simulink model "abs_EV"  (R2023a)
settings: Solver=ode45  StartTime=0  StopTime=15  FixedStep=0.002  RelTol=1e-3  AbsTol=1e-6
libraries: cstblocks x2, simulink x2, Solver_SF x1
settings Model: ExtModeTrigMode=oneshot  VariantFading=off  Creator=ywata  LastModifiedBy=USER
settings SolverCC: AutoScaleAbsTol=off  AlgebraicLoopSolver=TrustRegion
settings DataIOCC: SaveFormat=Array  SignalLoggingSaveFormat=ModelDataLogs  ReturnWorkspaceOutputs=off  SignalLoggingName=sigsOut
settings OptimizationCC: BlockReduction=off  BooleanDataType=off  ExpressionDepthLimit=2147483647  LifeSpan=inf
settings DebuggingCC: SaveWithParameterizedLinksMsg=none  UnderspecifiedInitializationDetection=Classic  MergeDetectMultiDrivingBlocksExec=none  SignalResolutionControl=TryResolveAllWithWarning  MultiTaskDSMMsg=warning  MultiTaskCondExecSysMsg=none  FcnCallInpInsideContextMsg=warning  UnconnectedInputMsg=warning  UnconnectedOutputMsg=warning  UnconnectedLineMsg=warning  StateNameClashWarn=warning  SFUnexpectedBacktrackingDiag=warning  SFNoUnconditionalDefaultTransitionDiag=warning  SFExecutionAtInitializationDiag=none  ArithmeticOperatorsInVariantConditions=warning
settings HardwareCC: ProdBitPerPointer=32  ProdBitPerSizeT=32  ProdBitPerPtrDiffT=32  ProdLargestAtomicFloat=None  ProdIntDivRoundTo=Undefined  ProdEndianess=Unspecified  ProdWordSize=32  ProdHWDeviceType=32-bit Generic  TargetUnknown=on
settings ModelReferenceCC: PropagateSignalLabelsOutOfModel=off
settings SFSimCC: SimUseLocalCustomCode=off  CustomCodeUndefinedFunction=UseInterfaceOnly
settings RTWCC: TemplateMakefile=grt_vc.tmf  RTWUseLocalCustomCode=off
settings CodeAppCC: StateflowObjectComments=on
settings GRTTargetCC: TargetFcnLib=ansi_tfl_tmw.mat  TargetLangStandard=C89/C90 (ANSI)  CombineOutputUpdateFcns=off  GRTInterface=on
settings ConfigComp: CovMetricSettings=dw  CovSaveCumulativeToWorkspaceVar=on  CovSaveSingleToWorkspaceVar=on  CovExternalEMLEnable=off

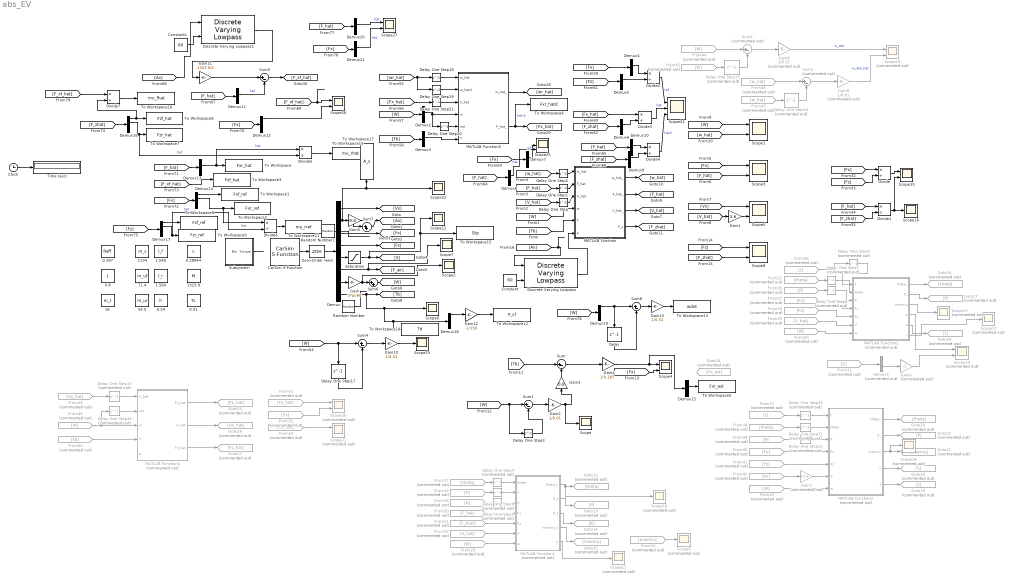
== system abs_EV ==
  0.01 : DataStoreMemory  DataStoreName=Ts  WriteAfterWriteMsg=warning  InitialValue=0.01  ShowAdditionalParam=off  OutDataTypeStr=double
  0.287 : DataStoreMemory  DataStoreName=Reff  WriteAfterWriteMsg=warning  InitialValue=0.287  ShowAdditionalParam=off  OutDataTypeStr=double
  0.28944 : DataStoreMemory  DataStoreName=c  WriteAfterWriteMsg=warning  InitialValue=0.29844  ShowAdditionalParam=off  OutDataTypeStr=double
  0.54 : DataStoreMemory  DataStoreName=h  WriteAfterWriteMsg=warning  InitialValue=0.54  ShowAdditionalParam=off  OutDataTypeStr=double
  0.8 : DataStoreMemory  DataStoreName=J  WriteAfterWriteMsg=warning  InitialValue=0.8  ShowAdditionalParam=off  OutDataTypeStr=double
  1.040 : DataStoreMemory  DataStoreName=l_f  WriteAfterWriteMsg=warning  InitialValue=1.040  ShowAdditionalParam=off  OutDataTypeStr=double
  1.560 : DataStoreMemory  DataStoreName=l_r  WriteAfterWriteMsg=warning  InitialValue=1.560  ShowAdditionalParam=off  OutDataTypeStr=double
  1134 : DataStoreMemory  DataStoreName=m_s  WriteAfterWriteMsg=warning  InitialValue=1134  ShowAdditionalParam=off  OutDataTypeStr=double
  1323.9 : DataStoreMemory  DataStoreName=M  WriteAfterWriteMsg=warning  InitialValue=1323.9  ShowAdditionalParam=off  OutDataTypeStr=double
  16 : DataStoreMemory  DataStoreName=m_t  WriteAfterWriteMsg=warning  InitialValue=16  ShowAdditionalParam=off  OutDataTypeStr=double
  54.5 : DataStoreMemory  DataStoreName=m_ur  WriteAfterWriteMsg=warning  InitialValue=54.5  ShowAdditionalParam=off  OutDataTypeStr=double
  71.4 : DataStoreMemory  DataStoreName=m_uf  WriteAfterWriteMsg=warning  InitialValue=71.4  ShowAdditionalParam=off  OutDataTypeStr=double
  CarSim S-Function : Solver_SF/CarSim S-Function  Priority=1  SIMFILE=simfile.sim  Run_RTs=off  vs_state_ind=Run  StopMode_ind=Vehicle Model
  Clock : Clock
  Constant : Constant  Value=60
  Constant1 : Constant  Value=60
  Delay : Delay  DelayLength=1  InitialCondition=67.655
  Delay One Step : Delay  DelayLength=1  InitialCondition=19.444
  Delay One Step1 : Delay  DelayLength=1  InitialCondition=[0 0 0 0]'
  Delay One Step10 : Delay  Commented=on  DelayLength=1
  Delay One Step11 : Delay  Commented=on  DelayLength=1  InitialCondition=[0 0]'
  Delay One Step12 : Delay  Commented=on  DelayLength=1  InitialCondition=[0 0;0 0]
  Delay One Step13 : Delay  Commented=on  DelayLength=1
  Delay One Step14 : Delay  Commented=on  DelayLength=1
  Delay One Step15 : Delay  Commented=on  DelayLength=1  InitialCondition=70/3.6
  Delay One Step16 : Delay  Commented=on  DelayLength=1  InitialCondition=67.75*ones(4,1)
  Delay One Step17 : Delay  DelayLength=1  InitialCondition=70/3.6/0.287
  Delay One Step18 : Delay  DelayLength=1  InitialCondition=67.655
  Delay One Step19 : Delay  InitialCondition=67.655
  Delay One Step2 : Delay  DelayLength=1  InitialCondition=[67.655 67.655 67.655 67.655]'
  Delay One Step20 : Delay  DelayLength=1  InitialCondition=67.655
  Delay One Step21 : Delay  DelayLength=1  InitialCondition=0
  Delay One Step3 : Delay  DelayLength=1  InitialCondition=[67.655 67.655 67.655 67.655]'
  Delay One Step4 : Delay  Commented=on  DelayLength=1  InitialCondition=ones(2,4)
  Delay One Step5 : Delay  Commented=on  DelayLength=1  InitialCondition=0.1*ones(2,4)
  Delay One Step6 : Delay  Commented=on  DelayLength=1  InitialCondition=0.1*ones(2,8)
  Delay One Step7 : Delay  Commented=on  DelayLength=1  InitialCondition=[300;0.1]
  Delay One Step8 : Delay  Commented=on  DelayLength=1  InitialCondition=[3 0;0 0.001]
  Delay One Step9 : Delay  Commented=on  DelayLength=1  InitialCondition=0
  Demux : Demux  Outputs=[1 1 4 4 4 1 4 4]
  Demux1 : Demux  Commented=on
  Demux{2..21} (20 alike) : Demux
  Discrete Varying Lowpass : cstblocks/Linear Parameter Varying/Discrete Varying Lowpass  N=1  w0=0  Ts=0.01
  Discrete Varying Lowpass1 : cstblocks/Linear Parameter Varying/Discrete Varying Lowpass  N=1  w0=0  Ts=0.01
  Divide{,1..7} (8 alike) : Product  Inputs=*/
  From17 : From  Commented=on  GotoTag=theta
  From18 : From  Commented=on  GotoTag=K
  From19 : From  Commented=on  GotoTag=P
  From20 : From  Commented=on  GotoTag=F_hat
  From21 : From  Commented=on  GotoTag=F_zhat
  From22 : From  Commented=on  GotoTag=V_hat
  From{23,30,43..45,49} (6 alike) : From  Commented=on  GotoTag=W
  From24 : From  Commented=on  GotoTag=maxmu
  From25 : From  Commented=on  GotoTag=theta
  From26 : From  Commented=on  GotoTag=P
  From27 : From  Commented=on  GotoTag=Fx
  From28 : From  Commented=on  GotoTag=Fz
  From29 : From  Commented=on  GotoTag=V_hat
  From31 : From  Commented=on  GotoTag=S
  From36 : From  Commented=on  GotoTag=t
  From37 : From  Commented=on  GotoTag=t
  From38 : From  Commented=on  GotoTag=theta
  From39 : From  Commented=on  GotoTag=P
  From40 : From  Commented=on  GotoTag=Fx
  From41 : From  Commented=on  GotoTag=Fz
  From42 : From  Commented=on  GotoTag=Vx
  From46 : From  Commented=on  GotoTag=w_hat
  From47 : From  Commented=on  GotoTag=w_hat
  From48 : From  Commented=on  GotoTag=Vx_hat
  From50 : From  Commented=on  GotoTag=Tb
  From51 : From  Commented=on  GotoTag=Fx_hat
  From52 : From  Commented=on  GotoTag=Fx
  From53 : From  Commented=on  GotoTag=Vx_hat
  Gain : Gain  Gain=2*pi/60
  Gain1 : Gain  Gain=3.6
  Gain10 : Gain  Gain=1/0.01
  Gain11 : Gain  Gain=1323.9/2
  Gain12 : Gain  Gain=-1/150
  Gain13 : Gain  Gain=1/0.01
  Gain2 : Gain  Gain=1/0.01
  Gain3 : Gain  Gain=0.8
  Gain4 : Gain  Gain=1/0.287
  Gain5 : Gain  Gain=9.8
  Gain6 : Gain  Commented=on  Gain=-1
  Gain7 : Gain  Commented=on  Gain=1/3.6
  Gain8 : Gain  Commented=on  Gain=1/0.01
  Gain9 : Gain  Commented=on  Gain=1/0.01
  Goto12 : Goto  Commented=on  GotoTag=theta
  Goto13 : Goto  Commented=on  GotoTag=P
  Goto14 : Goto  Commented=on  GotoTag=K
  Goto15 : Goto  Commented=on  GotoTag=maxmu
  Goto16 : Goto  Commented=on  GotoTag=theta
  Goto17 : Goto  Commented=on  GotoTag=P
  Goto18 : Goto  Commented=on  GotoTag=t
  Goto19 : Goto  Commented=on  GotoTag=t
  Goto20 : Goto  Commented=on  GotoTag=s
  Goto21 : Goto  Commented=on  GotoTag=maxmu
  Goto22 : Goto  Commented=on  GotoTag=P
  Goto23 : Goto  Commented=on  GotoTag=theta
  Goto24 : Goto  Commented=on  GotoTag=Fx_est
  Goto25 : Goto  Commented=on  GotoTag=Fx_hat
  Goto26 : Goto  Commented=on  GotoTag=Vx_hat
  Goto27 : Goto  Commented=on  GotoTag=Fz_hat
  MATLAB Function : MATLAB Function  TreatAsAtomicUnit=on
  MATLAB Function1 : MATLAB Function  Commented=on  TreatAsAtomicUnit=on
  MATLAB Function2 : MATLAB Function  Commented=on  TreatAsAtomicUnit=on
  MATLAB Function3 : MATLAB Function  Commented=on  TreatAsAtomicUnit=on
  MATLAB Function4 : MATLAB Function  Commented=on  TreatAsAtomicUnit=on
  MATLAB Function5 : MATLAB Function  TreatAsAtomicUnit=on
  Random Number : RandomNumber  Variance=0.01^2  SampleTime=0.01
  Random Number1 : RandomNumber  Variance=0.01  SampleTime=0.01
  Saturation : Saturate  UpperLimit=1  LowerLimit=-1
  Scope{,2,6..7,12,16,22..23} (8 alike) : Scope
  Scope{1,3..5,8,15,26..27} (8 alike) : Scope  NumInputPorts=2
  Scope{9..11,13,17..18} (6 alike) : Scope  Commented=on
  Scope{14,19..21} (4 alike) : Scope  Commented=on  NumInputPorts=2
  Scope24 : Scope  NumInputPorts=3
  Scope25 : Scope  NumInputPorts=3
  Subsystem : Subsystem
  Sum{,1,4..5,8} (5 alike) : Sum  Inputs=|+-
  Sum2 : Sum  Commented=on  Inputs=|+-
  Sum3 : Sum  Commented=on  Inputs=|+-
  Sum6 : Sum  Inputs=|++
  Sum7 : Sum  Inputs=|++
  Time (sec) : Display
      settings: Format=bank  Decimation=100
  To Workspace : ToWorkspace  VariableName=Fxr_hat  SaveFormat=Timeseries  SampleTime=-1
  To Workspace1 : ToWorkspace  VariableName=Fxf_ref  SaveFormat=Timeseries  SampleTime=-1
  To Workspace10 : ToWorkspace  VariableName=mu_rhat  SaveFormat=Timeseries  SampleTime=-1
  To Workspace11 : ToWorkspace  VariableName=mu_rref  SaveFormat=Timeseries  SampleTime=-1
  To Workspace12 : ToWorkspace  VariableName=P_cf  SaveFormat=Timeseries  SampleTime=-1
  To Workspace13 : ToWorkspace  VariableName=wdot  SaveFormat=Timeseries  SampleTime=-1
  To Workspace14 : ToWorkspace  VariableName=Td  SaveFormat=Timeseries  SampleTime=-1
  To Workspace15 : ToWorkspace  VariableName=Slip  SaveFormat=Timeseries  SampleTime=-1
  To Workspace16 : ToWorkspace  VariableName=mu_fhat  SaveFormat=Timeseries  SampleTime=-1
  To Workspace17 : ToWorkspace  VariableName=A_x  SaveFormat=Timeseries  SampleTime=-1
  To Workspace2 : ToWorkspace  VariableName=Fxr_ref  SaveFormat=Timeseries  SampleTime=-1
  To Workspace3 : ToWorkspace  VariableName=Fxf_hat  SaveFormat=Timeseries  SampleTime=-1
  To Workspace4 : ToWorkspace  VariableName=Fxr_hatd  SaveFormat=Timeseries  SampleTime=-1
  To Workspace5 : ToWorkspace  VariableName=Fxr_est  SaveFormat=Timeseries  SampleTime=-1
  To Workspace6 : ToWorkspace  VariableName=Fzf_hat  SaveFormat=Timeseries  SampleTime=-1
  To Workspace7 : ToWorkspace  VariableName=Fzr_hat  SaveFormat=Timeseries  SampleTime=-1
  To Workspace8 : ToWorkspace  VariableName=Fzf_ref  SaveFormat=Timeseries  SampleTime=-1
  To Workspace9 : ToWorkspace  VariableName=Fzr_ref  SaveFormat=Timeseries  SampleTime=-1
  Zero-Order Hold : ZeroOrderHold  SampleTime=0.01
  wires:
  CarSim S-Function/1 -> Zero-Order Hold/1
  Clock/1 -> Time (sec)/1
  Demux/1 -> [Vx]
  Demux/3 -> [Fx]
  Demux/4 -> [Fz]
  Demux/7 -> Gain/1
  Gain/1 -> Scope2/1, Sum6/1
  Demux/8 -> To Workspace14/1, Demux18/1, Scope6/1, [Tb]
  Zero-Order Hold/1 -> Demux/1
  [Tb] -> MATLAB Function/5(T)
  [W] -> MATLAB Function/4(w)
  MATLAB Function/3(V_hat_) -> [V_hat]
  MATLAB Function/2(F_hat_) -> [F_hat]
  MATLAB Function/1(w_hat_) -> [w_hat]
  [V_hat] -> Delay One Step/1
  Delay One Step/1 -> MATLAB Function/3(V_hat)
  [F_hat] -> Delay One Step1/1
  Delay One Step1/1 -> MATLAB Function/2(F_hat)
  [w_hat] -> Delay One Step2/1
  Delay One Step2/1 -> MATLAB Function/1(w_hat)
  [Fx] -> Scope3/1
  [F_hat] -> Scope3/2
  [V_hat] -> Gain1/1
  [Vx] -> Scope5/1
  Gain1/1 -> Scope5/2
  [W] -> Scope1/1
  [w_hat] -> Scope1/2
  [Tb] -> Sum/1
  [W] -> Delay One Step3/1, Sum1/1
  Delay One Step3/1 -> Sum1/2
  Gain2/1 -> Scope/1, Gain3/1
  Gain3/1 -> Sum/2
  Sum/1 -> Gain4/1
  Gain4/1 -> Demux15/1, Scope4/1
  [Fx] -> Scope4/2
  Sum1/1 -> Gain2/1
  Demux/6 -> Scope7/1, [F_air]
  MATLAB Function/4(F_z) -> [F_zhat]
  [F_zhat] -> Scope8/2
  [Fz] -> Scope8/1
  [Ax] -> Discrete Varying Lowpass/1
  Gain5/1 -> Sum7/1
  MATLAB Function1/1(theta_t) -> Scope10/1, Goto12/1
  MATLAB Function1/2(P_t) -> Goto13/1
  MATLAB Function1/3(K_t) -> Goto14/1
  MATLAB Function1/4(maxmu_t) -> Goto15/1
  From17/1 -> Delay One Step4/1
  Delay One Step4/1 -> MATLAB Function1/1(theta)
  From18/1 -> Delay One Step5/1
  Delay One Step5/1 -> MATLAB Function1/3(K)
  From19/1 -> Delay One Step6/1
  Delay One Step6/1 -> MATLAB Function1/2(P)
  From20/1 -> MATLAB Function1/4(Fx)
  From21/1 -> MATLAB Function1/5(Fz)
  From22/1 -> MATLAB Function1/6(V)
  From23/1 -> MATLAB Function1/7(w)
  From24/1 -> Scope9/1
  MATLAB Function1/5(s) -> Scope11/1
  From25/1 -> Delay One Step7/1
  Delay One Step7/1 -> MATLAB Function2/2(theta)
  Delay One Step8/1 -> MATLAB Function2/3(P)
  From26/1 -> Delay One Step8/1
  From27/1 -> MATLAB Function2/4(Fx)
  From28/1 -> MATLAB Function2/5(Fz)
  From30/1 -> MATLAB Function2/7(w)
  MATLAB Function2/1(theta_) -> Goto16/1
  MATLAB Function2/2(P_) -> Goto17/1
  MATLAB Function2/3(maxmu) -> Scope13/1
  MATLAB Function2/4(s) -> Scope14/1
  From31/1 -> Demux1/1
  Demux1/3 -> Gain6/1
  Gain6/1 -> Scope14/2
  [Fx] -> Divide/1
  [Fz] -> Divide/2
  Divide/1 -> Scope15/1
  [F_hat] -> Divide1/1
  [F_zhat] -> Divide1/2
  Divide1/1 -> Scope16/1, Scope15/2
  MATLAB Function2/5(t) -> Goto18/1
  From36/1 -> Delay One Step9/1
  Delay One Step9/1 -> MATLAB Function2/1("t ")
  MATLAB Function2/6(r) -> Scope17/1
  From29/1 -> MATLAB Function2/6(V)
  MATLAB Function3/5(t) -> Goto19/1
  MATLAB Function3/4(s) -> Goto20/1
  MATLAB Function3/3(maxmu) -> Scope18/1, Goto21/1
  MATLAB Function3/2(P_) -> Goto22/1
  MATLAB Function3/1(theta_) -> Goto23/1
  From37/1 -> Delay One Step10/1
  Delay One Step10/1 -> MATLAB Function3/1("t ")
  From38/1 -> Delay One Step11/1
  Delay One Step11/1 -> MATLAB Function3/2(theta)
  From39/1 -> Delay One Step12/1
  Delay One Step12/1 -> MATLAB Function3/3(P)
  From40/1 -> MATLAB Function3/4(Fx)
  From41/1 -> MATLAB Function3/5(Fz)
  From42/1 -> Gain7/1
  From43/1 -> MATLAB Function3/7(w)
  Gain7/1 -> MATLAB Function3/6(V)
  Demux/5 -> Saturation/1
  From44/1 -> Sum2/1
  From45/1 -> Delay One Step13/1
  Delay One Step13/1 -> Sum2/2
  Sum2/1 -> Gain8/1
  Gain8/1 -> Scope19/1  "w_dot"
  Gain9/1 -> Scope19/2  "w_dot_hat"
  From46/1 -> Sum3/1
  Sum3/1 -> Gain9/1
  From47/1 -> Delay One Step14/1
  Delay One Step14/1 -> Sum3/2
  MATLAB Function4/1(Fx_hat) -> Goto25/1
  MATLAB Function4/2(V_hat) -> Goto26/1
  MATLAB Function4/3(Fz_hat) -> Goto27/1
  From48/1 -> Delay One Step15/1
  Delay One Step15/1 -> MATLAB Function4/1("V_hat ")
  From49/1 -> Delay One Step16/1, MATLAB Function4/3(w)
  Delay One Step16/1 -> MATLAB Function4/2(wd)
  From50/1 -> MATLAB Function4/4(T)
  From51/1 -> Scope20/1
  From52/1 -> Scope20/2
  Saturation/1 -> To Workspace15/1, Scope12/1, [S]
  From53/1 -> Scope21/1
  [W] -> Delay One Step17/1, Sum4/1
  Delay One Step17/1 -> Sum4/2
  Sum4/1 -> Gain10/1
  Gain10/1 -> Scope23/1
  MATLAB Function5/1(w_hat_) -> [wr_hat]
  MATLAB Function5/2(F_hat_) -> To Workspace4/1, [Fx_hat]  "hat d"
  [wr_hat] -> Delay One Step19/1, Delay One Step18/1
  Delay One Step18/1 -> MATLAB Function5/1(w_hat)
  Delay One Step19/1 -> MATLAB Function5/2(w_hatd)
  [Fx_hat] -> Delay One Step21/1
  [W] -> Demux2/1
  Demux2/2 -> Delay One Step20/1, MATLAB Function5/4(w)
  Delay One Step20/1 -> MATLAB Function5/5(wd)
  [Tb] -> Demux3/1
  Demux3/2 -> MATLAB Function5/6(T)
  [Fx_hat] -> Divide3/1
  [Fx] -> Demux4/1
  Delay One Step21/1 -> MATLAB Function5/3(F_hat)
  [Fz] -> Demux5/1
  Demux4/2 -> Divide2/1
  Demux5/2 -> Divide2/2
  Divide2/1 -> Scope24/1  "ref"
  [F_zhat] -> Demux6/1
  Demux6/2 -> Divide3/2
  Divide3/1 -> Scope24/2  "hat"
  [Fx] -> Demux7/1
  Demux7/2 -> Scope25/2  "ref"
  [F_hat] -> Demux8/1
  Demux8/2 -> Scope25/3  "hat"
  [F_hat] -> Demux10/1
  Demux9/2 -> Divide4/2
  [F_zhat] -> Demux9/1
  Demux10/2 -> Divide4/1
  Divide4/1 -> Scope24/3  "hat2"
  [F_hat] -> Demux11/1
  Demux11/2 -> Sum5/2  "hat"
  [Ax] -> Discrete Varying Lowpass1/1
  Gain11/1 -> Sum5/1
  Sum5/1 -> [F_xf_hat]
  [F_xf_hat] -> Scope26/1
  [Fx] -> Demux12/1
  Demux12/1 -> Scope26/2
  [F_hat] -> Demux13/1
  Demux13/2 -> Divide5/1, To Workspace/1  "hat"
  [Fx] -> Demux14/1
  Demux14/1 -> To Workspace1/1
  Demux14/2 -> Divide6/1, To Workspace2/1  "hat"
  [F_xf_hat] -> To Workspace3/1
  Demux15/2 -> To Workspace5/1
  Sum6/1 -> [W]
  Random Number/1 -> ?
  Demux/2 -> Scope22/1, To Workspace17/1, Gain5/1
  Constant/1 -> Discrete Varying Lowpass/2
  Discrete Varying Lowpass/1 -> MATLAB Function/6(a)
  [F_zhat] -> Demux16/1
  Demux16/1 -> Divide7/2, To Workspace6/1
  Demux16/2 -> Divide5/2, To Workspace7/1  "hat"
  [Fz] -> Demux17/1
  Demux17/1 -> To Workspace8/1
  Demux17/2 -> Divide6/2, To Workspace9/1  "hat"
  Random Number1/1 -> ?
  Sum7/1 -> [Ax]
  Constant1/1 -> Discrete Varying Lowpass1/2
  Discrete Varying Lowpass1/1 -> Gain11/1
  Divide5/1 -> To Workspace10/1
  Divide6/1 -> To Workspace11/1
  Demux18/1 -> Gain12/1
  Gain12/1 -> To Workspace12/1
  [W] -> Demux19/1
  Demux19/1 -> Delay/1, Sum8/1
  Delay/1 -> Sum8/2
  Sum8/1 -> Gain13/1
  Gain13/1 -> To Workspace13/1
  Subsystem/1(Brk. Torque) -> ?
  Demux20/2 -> Scope27/1  "hat"
  [F_hat] -> Demux20/1
  [Fx] -> Demux21/1
  Demux21/2 -> Scope27/2  "hat"
  [F_xf_hat] -> Divide7/1
  Divide7/1 -> To Workspace16/1

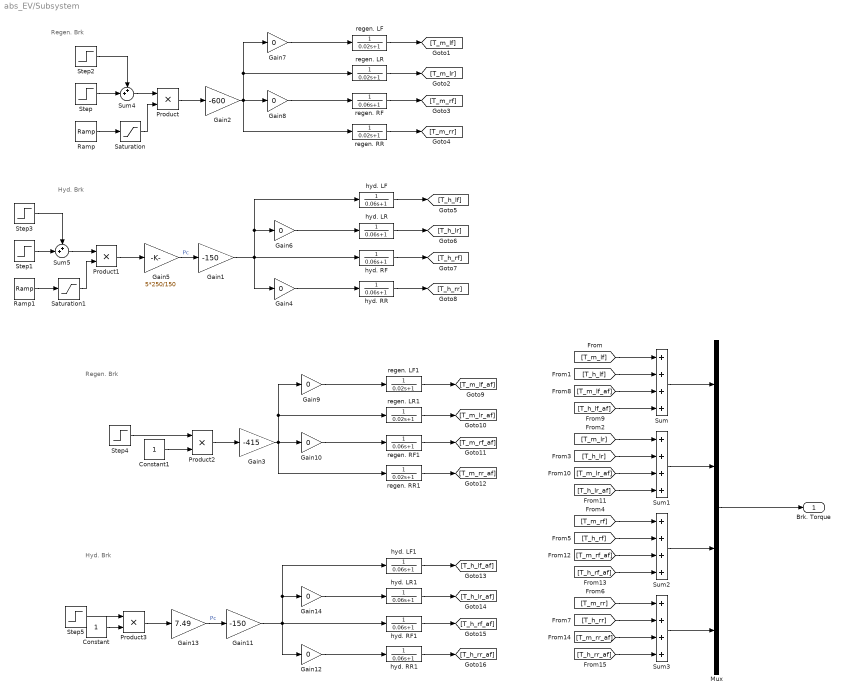
== system abs_EV/Subsystem ==
  note: Regen. Brk
  note: Hyd. Brk
  note: Regen. Brk
  note: Hyd. Brk
  Constant : Constant
  Constant1 : Constant
  Gain1 : Gain  Gain=-150
  Gain{4,6..10,12,14} (8 alike) : Gain  Gain=0
  Gain11 : Gain  Gain=-150
  Gain13 : Gain  Gain=7.49
  Gain2 : Gain  Gain=-600
  Gain3 : Gain  Gain=-415
  Gain5 : Gain  Gain=5*250/150
  Mux : Mux
  Product{,1..3} (4 alike) : Product
  Ramp : simulink/Sources/Ramp  slope=1/0.3  start=3  InitialOutput=0
  Ramp1 : simulink/Sources/Ramp  slope=1/0.3  start=3  InitialOutput=0
  Saturation : Saturate  UpperLimit=1  LowerLimit=0
  Saturation1 : Saturate  UpperLimit=1  LowerLimit=0
  Step : Step  Time=3  SampleTime=0.01
  Step1 : Step  Time=3  SampleTime=0.01
  Step2 : Step  Time=3.32  After=-1  SampleTime=0.01
  Step3 : Step  Time=3.32  After=-1  SampleTime=0.01
  Step4 : Step  Time=3.32  SampleTime=0.01
  Step5 : Step  Time=3.32  SampleTime=0.01
  Sum{,1..3} (4 alike) : Sum  Inputs=++++
  Sum4 : Sum  Inputs=++|
  Sum5 : Sum  Inputs=++|
  hyd. LF : TransferFcn  Denominator=[0.06 1]
  hyd. LF1 : TransferFcn  Denominator=[0.06 1]
  hyd. LR : TransferFcn  Denominator=[0.06 1]
  hyd. LR1 : TransferFcn  Denominator=[0.06 1]
  hyd. RF : TransferFcn  Denominator=[0.06 1]
  hyd. RF1 : TransferFcn  Denominator=[0.06 1]
  hyd. RR : TransferFcn  Denominator=[0.06 1]
  hyd. RR1 : TransferFcn  Denominator=[0.06 1]
  regen. LF : TransferFcn  Denominator=[0.02 1]
  regen. LF1 : TransferFcn  Denominator=[0.02 1]
  regen. LR : TransferFcn  Denominator=[0.02 1]
  regen. LR1 : TransferFcn  Denominator=[0.02 1]
  regen. RF : TransferFcn  Denominator=[0.06 1]
  regen. RF1 : TransferFcn  Denominator=[0.06 1]
  regen. RR : TransferFcn  Denominator=[0.02 1]
  regen. RR1 : TransferFcn  Denominator=[0.02 1]
  Brk. Torque : Outport
  wires:
  Saturation/1 -> Product/2
  Product/1 -> Gain2/1
  Ramp/1 -> Saturation/1
  Gain2/1 -> regen. RR/1, regen. LR/1, Gain7/1, Gain8/1
  regen. LF/1 -> [T_m_lf]
  regen. LR/1 -> [T_m_lr]
  regen. RF/1 -> [T_m_rf]
  regen. RR/1 -> [T_m_rr]
  Ramp1/1 -> Saturation1/1
  Product1/1 -> Gain5/1
  Saturation1/1 -> Product1/2
  hyd. RF/1 -> [T_h_rf]
  hyd. RR/1 -> [T_h_rr]
  hyd. LR/1 -> [T_h_lr]
  Gain6/1 -> hyd. LR/1
  Gain4/1 -> hyd. RR/1
  hyd. LF/1 -> [T_h_lf]
  Sum/1 -> Mux/1
  [T_m_lf] -> Sum/1
  [T_h_lf] -> Sum/2
  Mux/1 -> Brk. Torque/1
  Gain7/1 -> regen. LF/1
  Gain8/1 -> regen. RF/1
  Gain1/1 -> hyd. RF/1, hyd. LF/1, Gain6/1, Gain4/1
  Gain5/1 -> Gain1/1  "Pc"
  Step/1 -> Sum4/2
  Sum4/1 -> Product/1
  Step2/1 -> Sum4/1
  Step3/1 -> Sum5/1
  Step1/1 -> Sum5/2
  Sum5/1 -> Product1/1
  Step4/1 -> Product2/1
  Gain10/1 -> regen. RF1/1
  Gain3/1 -> regen. RR1/1, regen. LR1/1, Gain9/1, Gain10/1
  regen. LR1/1 -> [T_m_lr_af]
  regen. RF1/1 -> [T_m_rf_af]
  regen. LF1/1 -> [T_m_lf_af]
  Gain9/1 -> regen. LF1/1
  Product2/1 -> Gain3/1
  regen. RR1/1 -> [T_m_rr_af]
  Gain13/1 -> Gain11/1  "Pc"
  Gain11/1 -> hyd. RF1/1, hyd. LF1/1, Gain14/1, Gain12/1
  hyd. LF1/1 -> [T_h_lf_af]
  Gain12/1 -> hyd. RR1/1
  Product3/1 -> Gain13/1
  hyd. LR1/1 -> [T_h_lr_af]
  hyd. RF1/1 -> [T_h_rf_af]
  hyd. RR1/1 -> [T_h_rr_af]
  Gain14/1 -> hyd. LR1/1
  Step5/1 -> Product3/1
  [T_m_lf_af] -> Sum/3
  [T_h_lf_af] -> Sum/4
  [T_m_lr_af] -> Sum1/3
  [T_m_lr] -> Sum1/1
  [T_h_lr_af] -> Sum1/4
  [T_h_lr] -> Sum1/2
  Sum1/1 -> Mux/2
  [T_m_rf_af] -> Sum2/3
  [T_m_rf] -> Sum2/1
  [T_h_rf_af] -> Sum2/4
  [T_h_rf] -> Sum2/2
  Sum2/1 -> Mux/3
  [T_m_rr_af] -> Sum3/3
  [T_m_rr] -> Sum3/1
  [T_h_rr_af] -> Sum3/4
  [T_h_rr] -> Sum3/2
  Sum3/1 -> Mux/4
  Constant/1 -> Product3/2
  Constant1/1 -> Product2/2

== matlab function abs_EV/MATLAB Function3 ==
  data: t input; theta input; theta_ output; P input; Fx input; Fz input; V input; w input; P_ output; maxmu output; s output; Reff data_store_memory; t output; Ts data_store_memory
function [theta_,P_,maxmu,s,t]   = fcn(t,theta,P,Fx,Fz,V,w)

global Reff Ts;
% theta_t = zeros(2,4); P_t = zeros(2,8); K_t = zeros(2,4); maxmu_t = zeros(1,4);
Q = [100 0;0 0.01]; R = 10;
if t<3 || t>5
    t = t + Ts;
    theta_ = [0;0]; P_ = [30 0;0 0.01]; maxmu = 0; s = (V-Reff*w(3))/V;
else
    
    for i = 1:1
        s = (V-Reff*w(i))/V;
        F = eye(2);
        H = [((s-theta(2))^3+theta(2)^3)/3 -theta(1)*(s-theta(2))^2+theta(1)*theta(2)^2];
        Pm = F*P*F'+Q;
        K = Pm*H'*(H*Pm*H'+R);
        yhat = theta(1)/3*(s-theta(2))^3 + 1/3*theta(1)*theta(2)^3;
        theta_ = theta + K*(-Fx(i)/Fz(i)-yhat);
        P_ = (eye(2)-K*H)*Pm;
        
        maxmu = 1/3*theta_(1)*theta_(2)^3;
        t = t + Ts;
    end
end
end

== matlab function abs_EV/MATLAB Function4 ==
  data: V_hat input; wd input; Fx_hat output; w input; T input; V_hat output; c data_store_memory; Reff data_store_memory; J data_store_memory; M data_store_memory; Ts data_store_memory; m_s data_store_memory; m_uf data_store_memory; m_ur data_store_memory; m_t data_store_memory; l_f data_store_memory; l_r data_store_memory; h data_store_memory; Fz_hat output; a input
function [Fx_hat,V_hat,Fz_hat]  = fcn(V_hat,wd,w,T,a)

global c Reff J M Ts m_s m_uf m_ur m_t l_f l_r h;

Fx_hat = 1/Reff*(T-J*(w-wd)/Ts);

V_hat = V_hat + (sum(Fx_hat) - c*V_hat^2)/M*Ts;

F_zf = ((m_s*l_r + (m_uf + 2*m_t)*(l_f + l_r))*9.8 - m_s*h*a-c*V_hat^2*h)/(2*(l_f+l_r));
F_zr = ((m_s*l_f + (m_ur + 2*m_t)*(l_f + l_r))*9.8 + m_s*h*a-c*V_hat^2*h)/(2*(l_f+l_r));

Fz_hat = [F_zf F_zr F_zf F_zr]';
end

== matlab function abs_EV/MATLAB Function5 ==
  data: w_hat input; w_hatd input; w_hat_ output; F_hat input; w input; wd input; T input; F_hat_ output; c data_store_memory; Reff data_store_memory; J data_store_memory; M data_store_memory; Ts data_store_memory; m_s data_store_memory; m_uf data_store_memory; m_ur data_store_memory; m_t data_store_memory; l_f data_store_memory; l_r data_store_memory; h data_store_memory
function [w_hat_,F_hat_]  = fcn(w_hat,w_hatd,F_hat,w,wd,T)

global Reff J Ts;
l1 = 1; l2 = 1000; l3 = 100;

w_hatdot = 1/J*T - Reff/J*F_hat + l1*(w-w_hat);
w_hat_ = w_hat + w_hatdot*Ts;

F_xhatdot = -l2*(w-w_hat) - l3*((w-wd)/Ts - (w_hat-w_hatd)/Ts);
F_hat_ = F_hat + F_xhatdot*Ts;




end

== matlab function abs_EV/MATLAB Function1 ==
  data: theta input; P input; K input; Fx input; theta_t output; Fz input; V input; w input; P_t output; K_t output; c data_store_memory; Reff data_store_memory; J data_store_memory; M data_store_memory; Ts data_store_memory; m_s data_store_memory; m_uf data_store_memory; m_ur data_store_memory; m_t data_store_memory; l_f data_store_memory; l_r data_store_memory; h data_store_memory; maxmu_t output; s output
function [theta_t,P_t,K_t,maxmu_t,s]  = fcn(theta,P,K,Fx,Fz,V,w)

global Reff;
theta_t = zeros(2,4); P_t = zeros(2,8); K_t = zeros(2,4); maxmu_t = zeros(1,4);
for i = 1:4
    s = (V-Reff*w(i))/V;
    F = [((s-theta(2,i))^3+theta(2,i)^3)/3 -theta(1,i)*(s-theta(2,i))^2+theta(1,i)*theta(2,i)^2];
    yhat = F*theta(:,i);
    theta_ = theta(:,i) + K(:,i)*(yhat-Fx(i)/Fz(i));
    P_ = 1/0.95*(P(:,2*i-1:2*i)-P(:,2*i-1:2*i)*F'*F*P(:,2*i-1:2*i)/(0.95+F*P(:,2*i-1:2*i)*F'));
    K_ = P(:,2*i-1:2*i)*F'/(0.95+F*P(:,2*i-1:2*i)*F');
    
    maxmu = 1/3*theta_(1)*theta_(2)^3;

    theta_t(:,i) = theta_;
    P_t(:,2*i-1:2*i) = P_;
    K_t(:,i) = K_;
    maxmu_t(i) = maxmu;
end
end

== matlab function abs_EV/MATLAB Function ==
  data: w_hat input; w_hat_ output; F_hat input; V_hat input; w input; T input; F_hat_ output; V_hat_ output; c data_store_memory; Reff data_store_memory; J data_store_memory; M data_store_memory; Ts data_store_memory; m_s data_store_memory; m_uf data_store_memory; m_ur data_store_memory; m_t data_store_memory; l_f data_store_memory; l_r data_store_memory; h data_store_memory; F_z output; a input
function [w_hat_,F_hat_,V_hat_,F_z]  = fcn(w_hat,F_hat,V_hat,w,T,a)

global c Reff J M Ts m_s m_uf m_ur m_t l_f l_r h;
l1 = 100; l2 = -8000;
X = [w_hat(1),F_hat(1),w_hat(2),F_hat(2),w_hat(3),F_hat(3),w_hat(4),F_hat(4),V_hat]';
U = [T(1)/J,0,T(2)/J,0,T(3)/J,0,T(4)/J,0,-c/M*V_hat^2]';
Y = [w(1), 0, w(2), 0, w(3), 0, w(4), 0, 0]';

A = [0 -Reff/J zeros(1,7); zeros(1,9); zeros(1,2) 0 -Reff/J zeros(1,5); zeros(1,9); zeros(1,4) 0 -Reff/J zeros(1,3); zeros(1,9); zeros(1,6) 0 -Reff/J 0; zeros(1,9); 0 1/M 0 1/M 0 1/M 0 1/M 0];
B = eye(9);
C = [1 0 zeros(1,7); zeros(1,9); zeros(1,2) 1 0 zeros(1,5); zeros(1,9); zeros(1,4) 1 0 zeros(1,3); zeros(1,9); zeros(1,6) 1 0 zeros(1,1); zeros(1,9); zeros(1,9);];
L0 = [l1 0;l2 0]; L = [L0 zeros(2,7); zeros(2,2) L0 zeros(2,5); zeros(2,4) L0 zeros(2,3); zeros(2,6) L0 zeros(2,1); zeros(1,9)];
X_ = (eye(9)+A*Ts)*X + Ts*B*U + Ts*L*(Y-C*X);

w_hat_ = X_([1,3,5,7]); F_hat_ = X_([2,4,6,8]); V_hat_ = X_(9);

%Fz
F_zf = ((m_s*l_r + (m_uf + 2*m_t)*(l_f + l_r))*9.8 - m_s*h*a)/(2*(l_f+l_r));
F_zr = ((m_s*l_f + (m_ur + 2*m_t)*(l_f + l_r))*9.8 + m_s*h*a)/(2*(l_f+l_r));

F_z = [F_zf F_zr F_zf F_zr]';
end

== matlab function abs_EV/MATLAB Function2 ==
  data: t input; theta input; theta_ output; P input; Fx input; Fz input; V input; w input; P_ output; maxmu output; s output; Reff data_store_memory; t output; Ts data_store_memory; r output
function [theta_,P_,maxmu,s,t,r]   = fcn(t,  theta,P,Fx,Fz,V,w)

global Reff Ts;
% theta_t = zeros(2,4); P_t = zeros(2,8); K_t = zeros(2,4); maxmu_t = zeros(1,4);
if t<3 || t>3.3
    t = t + Ts;
    theta_ = [3000;0.1]; P_ = [100 0;0 0.1]; maxmu = 0; s = (V-Reff*w(3))/V; r = 0;
else
    

    for i = 3:3
        ff = 0.915;
        s = (V-Reff*w(i))/V;
        F = [((s-theta(2))^3+theta(2)^3)/3 -theta(1)*(s-theta(2))^2+theta(1)*theta(2)^2];
        yhat = theta(1)/3*(s-theta(2))^3 + 1/3*theta(1)*theta(2)^3;
        % yhat = F*theta;
        P_ = 1/ff*(P-P*F'*F*P/(ff+F*P*F'));
        K_ = P*F'/(ff+F*P*F');
        r = -Fx(i)/Fz(i)-yhat;
        theta_ = theta + K_*(r);
        
        maxmu = 1/3*theta_(1)*theta_(2)^3;
        t = t + Ts;
    end
end
end
